simulink model "VCUSTM32"  (R2024b)
settings: Solver=FixedStepDiscrete  StartTime=0.0  StopTime=1  FixedStep=0.001  RelTol=1e-3  EnableMultiTasking=on
libraries: stm32blockslib x16, simulink x4, canmsglib x3, stm32f4xxblockslib x2, stm32h7xxblockslib x1
settings Model: STM32="{\"DigitalPortRead\":[{\"ID\":\"CANTestingSTM32:620\"},{\"ID\":\"VCUSTM32:620\"}],\"SPIControllerTransfer\":[{\"ID\":\"CANTestingSTM32:616\"},{\"ID\":\"CANTestingSTM32:631\"},{\"ID\":\"CANTestingSTM32:632\"},{\"ID\":\"CANTestingSTM32:633\"},{\"ID\":\"CANTestingSTM32:634\"},{\"ID\":\"CANTestingSTM32:635\"},{\"ID\":\"CANTestingSTM32:636\"},{\"ID\":\"CANTestingSTM32:637\"},{\"ID\":\"CANTestingSTM32:638\"},{\"ID\":\"CANTestingSTM32:653\"},{\"ID\":\"CANTestingSTM32:709\"},{\"ID\":\"CANTestingSTM32:716\"},{\"ID\":\"CANTestingSTM32:722\"},{\"ID\":\"CANTestingSTM32:728\"},{\"ID\":\"CANTestingSTM32:786\"},{\"ID\":\"CANTestingSTM32:787\"}],\"AnalogInputForH7\":[{\"ID\":\"CANTestingSTM32:731\"},{\"ID\":\"VCUSTM32:731\"}],\"DigitalPortWrite\":[{\"ID\":\"CANTestingSTM32:747\"},{\"ID\":\"VCUSTM32:747\"}]}"  Creator=will  LastModifiedBy=William
settings SolverCC: AlgebraicLoopSolver=TrustRegion
settings DataIOCC: ReturnWorkspaceOutputs=off
settings OptimizationCC: DefaultParameterBehavior=Inlined  EnhancedBackFolding=on  PassReuseOutputArgsAs=Individual arguments  ZeroExternalMemoryAtStartup=off  ZeroInternalMemoryAtStartup=off  MaxStackSize=512  OptimizeBlockOrder=speed  DifferentSizesBufferReuse=on  OptimizationCustomize=off  EfficientTunableParamExpr=on
settings DebuggingCC: ParameterTunabilityLossMsg=error  UnconnectedInputMsg=warning  UnconnectedOutputMsg=warning  UnconnectedLineMsg=warning  ArithmeticOperatorsInVariantConditions=warning
settings HardwareCC: ProdBitPerPointer=32  ProdBitPerSizeT=32  ProdBitPerPtrDiffT=32  ProdLargestAtomicInteger=Long  ProdLargestAtomicFloat=Double  ProdWordSize=32  ProdLongLongMode=on  ProdHWDeviceType=ARM Compatible->ARM Cortex-M
settings ModelReferenceCC: EnableRefExpFcnMdlSchedulingChecks=on
settings SFSimCC: MATLABDynamicMemAlloc=off  CustomCodeUndefinedFunction=UseInterfaceOnly
settings RTWCC: Description=Embedded Coder  SystemTargetFile=ert.tlc  HardwareBoard=STM32H7xx Based (Single-core)  TemplateMakefile=ert_default_tmf  CustomHeaderCode="#include \"stm32h7xx_ll_tim.h\""  CustomInitializer=LL_TIM_EnableCounter(TIM2);  Toolchain=GNU Tools for ARM Embedded Processors  GPUComputeCapability=3.5
settings CodeAppCC: ForceParamTrailComments=on  IgnoreCustomStorageClasses=off  OperatorAnnotations=on  SimulinkDataObjDesc=on  SFDataObjDesc=on  InsertBlockDesc=on
settings ERTTargetCC: TargetLangStandard=C99 (ISO)  CodeReplacementLibrary=ARM Cortex-M  ExtModeTransport=3  ExtModeStaticAlloc=on  ExtModeStaticAllocSize=2048  ExtModeMexFile=ext_xcp  ExtModeIntrfLevel=Level2 - Open

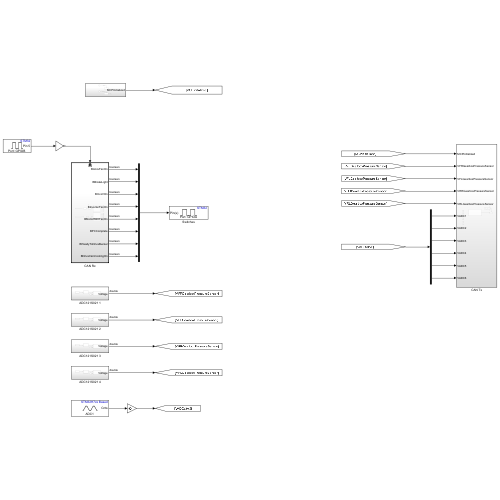
[thumbnail: Simulink's stored preview of the top-level diagram]
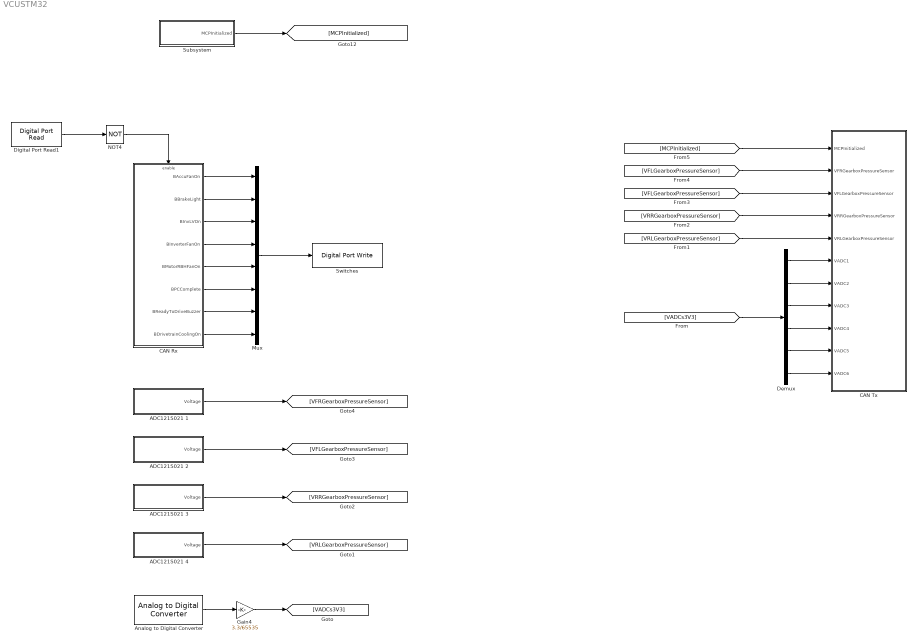
== system VCUSTM32 ==
  ADC121S021 1 : Subsystem
  ADC121S021 2 : Subsystem
  ADC121S021 3 : Subsystem
  ADC121S021 4 : Subsystem
  Analog to Digital Converter : stm32h7xxblockslib/Analog to Digital Converter  ADCModule=ADC1  ConversionGroup=Regular  TriggerMode=Trigger and read  NumberOfConversions=6  EnableBufferConv=off  BufferLength=1  OutputStatus=off  SampleTime=-1  EnableSimPort=off  hoistedMaskSrc=ECSoC/ECSimCodegen/Analog to Digital Converter
  CAN Rx : Subsystem  TreatAsAtomicUnit=on
  CAN Tx : Subsystem
  Demux : Demux  Outputs=6
  Digital Port Read1 : stm32f4xxblockslib/Digital Port Read  PortName=GPIOB  PinNumber=5  ReadOperation=on  IOAsArray=off  SampleTime=-1  EnableSimPort=off  hoistedMaskSrc=ECSoC/ECSimCodegen/Digital Port Read
      settings: LibrarySourceBlock=stm32f2xxblockslib/Digital Port Read
  Gain4 : Gain  Gain=3.3/65535  OutDataTypeStr=single
  Mux : Mux  Inputs=8
  NOT4 : Logic  Operator=NOT  IconShape=distinctive  AllPortsSameDT=off  OutDataTypeStr=boolean
  Subsystem : Subsystem
  Switches : stm32f4xxblockslib/Digital Port Write  PortName=GPIOA  PinNumber=[0, 1, 2, 3, 4]  ReadOperation=off  IOAsArray=on  EnableSimPort=off  hoistedMaskSrc=ECSoC/ECSimCodegen/Digital Port Write
      settings: LibrarySourceBlock=stm32h7xxblockslib/Digital Port Write
  wires:
  Subsystem/1(MCPInitialized) -> [MCPInitialized]
  NOT4/1 -> CAN Rx/Enable
  Digital Port Read1/1 -> NOT4/1
  Analog to Digital Converter/1 -> Gain4/1
  CAN Rx/6(BPCComplete) -> Mux/6
  CAN Rx/5(BMotorRBHFanOn) -> Mux/5
  CAN Rx/4(BInverterFanOn) -> Mux/4
  CAN Rx/3(BInvLVOn) -> Mux/3
  CAN Rx/2(BBrakeLight) -> Mux/2
  CAN Rx/1(BAccuFanOn) -> Mux/1
  CAN Rx/7(BReadyToDriveBuzzer) -> Mux/7
  CAN Rx/8(BDrivetrainCoolingOn) -> Mux/8
  Mux/1 -> Switches/1
  Gain4/1 -> [VADCs3V3]
  Demux/6 -> CAN Tx/11(VADC6)
  Demux/5 -> CAN Tx/10(VADC5)
  Demux/4 -> CAN Tx/9(VADC4)
  Demux/3 -> CAN Tx/8(VADC3)
  Demux/2 -> CAN Tx/7(VADC2)
  Demux/1 -> CAN Tx/6(VADC1)
  [VADCs3V3] -> Demux/1
  ADC121S021 1/1(Voltage) -> [VFRGearboxPressureSensor]
  ADC121S021 2/1(Voltage) -> [VFLGearboxPressureSensor]
  ADC121S021 3/1(Voltage) -> [VRRGearboxPressureSensor]
  ADC121S021 4/1(Voltage) -> [VRLGearboxPressureSensor]
  [VFLGearboxPressureSensor] -> CAN Tx/2(VFRGearboxPressureSensor)
  [VFLGearboxPressureSensor] -> CAN Tx/3(VFLGearboxPressureSensor)
  [VRRGearboxPressureSensor] -> CAN Tx/4(VRRGearboxPressureSensor)
  [VRLGearboxPressureSensor] -> CAN Tx/5(VRLGearboxPressureSensor)
  [MCPInitialized] -> CAN Tx/1(MCPInitialized)

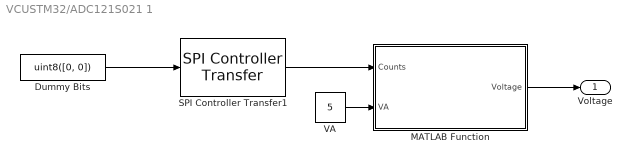
== system VCUSTM32/ADC121S021 1 ==
  Dummy Bits : Constant  Value=uint8([0, 0])
  MATLAB Function : MATLAB Function  TreatAsAtomicUnit=on
  SPI Controller Transfer1 : stm32blockslib/SPI Controller Transfer  Priority=2  SPIModuleSelect=SPI1  ClockPolarity=Low  ClockPhase=1 Edge  SPIModule=uint32(0)  Mode=Master  BusSpeed=uint32(1000000)  FirstBitToTransfer=Most significant bit (MSB)  ClockMode=0  BlockFunction=Transfer  EnableRegisterAddress=off  RegisterAddress=0  OutputDataType=uint8  OutputDataLength=1  OutputStatus=off  BlockingMode=on  Timeout=0.01  DataBits=8  UseCustomSSPin=Explicit GPIO calls  ActiveLowSSPin=Active low  Port_Select=GPIOA  Pin=4
      settings: LibrarySourceBlock=stm32h7xxblockslib/SPI Controller Transfer
  VA : Constant  Value=5
  Voltage : Outport  OutDataTypeStr=double
  wires:
  Dummy Bits/1 -> SPI Controller Transfer1/1
  SPI Controller Transfer1/1 -> MATLAB Function/1(Counts)
  VA/1 -> MATLAB Function/2(VA)
  MATLAB Function/1(Voltage) -> Voltage/1

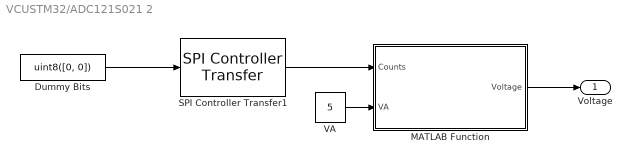
== system VCUSTM32/ADC121S021 2 ==
  Dummy Bits : Constant  Value=uint8([0, 0])
  MATLAB Function : MATLAB Function  TreatAsAtomicUnit=on
  SPI Controller Transfer1 : stm32blockslib/SPI Controller Transfer  Priority=2  SPIModuleSelect=SPI1  ClockPolarity=Low  ClockPhase=1 Edge  SPIModule=uint32(0)  Mode=Master  BusSpeed=uint32(1000000)  FirstBitToTransfer=Most significant bit (MSB)  ClockMode=0  BlockFunction=Transfer  EnableRegisterAddress=off  RegisterAddress=0  OutputDataType=uint8  OutputDataLength=1  OutputStatus=off  BlockingMode=on  Timeout=0.01  DataBits=8  UseCustomSSPin=Explicit GPIO calls  ActiveLowSSPin=Active low  Port_Select=GPIOA  Pin=4
      settings: LibrarySourceBlock=stm32h7xxblockslib/SPI Controller Transfer
  VA : Constant  Value=5
  Voltage : Outport  OutDataTypeStr=double
  wires:
  Dummy Bits/1 -> SPI Controller Transfer1/1
  SPI Controller Transfer1/1 -> MATLAB Function/1(Counts)
  VA/1 -> MATLAB Function/2(VA)
  MATLAB Function/1(Voltage) -> Voltage/1

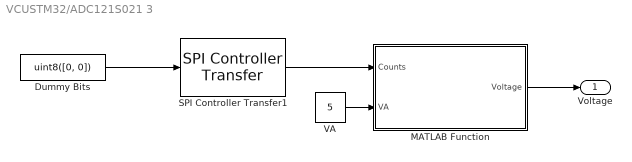
== system VCUSTM32/ADC121S021 3 ==
  Dummy Bits : Constant  Value=uint8([0, 0])
  MATLAB Function : MATLAB Function  TreatAsAtomicUnit=on
  SPI Controller Transfer1 : stm32blockslib/SPI Controller Transfer  Priority=2  SPIModuleSelect=SPI1  ClockPolarity=Low  ClockPhase=1 Edge  SPIModule=uint32(0)  Mode=Master  BusSpeed=uint32(1000000)  FirstBitToTransfer=Most significant bit (MSB)  ClockMode=0  BlockFunction=Transfer  EnableRegisterAddress=off  RegisterAddress=0  OutputDataType=uint8  OutputDataLength=1  OutputStatus=off  BlockingMode=on  Timeout=0.01  DataBits=8  UseCustomSSPin=Explicit GPIO calls  ActiveLowSSPin=Active low  Port_Select=GPIOA  Pin=4
      settings: LibrarySourceBlock=stm32h7xxblockslib/SPI Controller Transfer
  VA : Constant  Value=5
  Voltage : Outport  OutDataTypeStr=double
  wires:
  Dummy Bits/1 -> SPI Controller Transfer1/1
  SPI Controller Transfer1/1 -> MATLAB Function/1(Counts)
  VA/1 -> MATLAB Function/2(VA)
  MATLAB Function/1(Voltage) -> Voltage/1

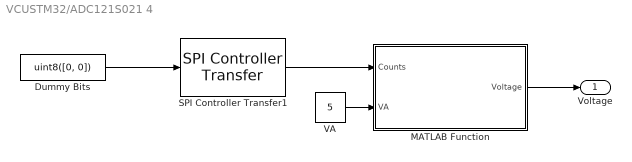
== system VCUSTM32/ADC121S021 4 ==
  Dummy Bits : Constant  Value=uint8([0, 0])
  MATLAB Function : MATLAB Function  TreatAsAtomicUnit=on
  SPI Controller Transfer1 : stm32blockslib/SPI Controller Transfer  Priority=2  SPIModuleSelect=SPI1  ClockPolarity=Low  ClockPhase=1 Edge  SPIModule=uint32(0)  Mode=Master  BusSpeed=uint32(1000000)  FirstBitToTransfer=Most significant bit (MSB)  ClockMode=0  BlockFunction=Transfer  EnableRegisterAddress=off  RegisterAddress=0  OutputDataType=uint8  OutputDataLength=1  OutputStatus=off  BlockingMode=on  Timeout=0.01  DataBits=8  UseCustomSSPin=Explicit GPIO calls  ActiveLowSSPin=Active low  Port_Select=GPIOA  Pin=4
      settings: LibrarySourceBlock=stm32h7xxblockslib/SPI Controller Transfer
  VA : Constant  Value=5
  Voltage : Outport  OutDataTypeStr=double
  wires:
  Dummy Bits/1 -> SPI Controller Transfer1/1
  SPI Controller Transfer1/1 -> MATLAB Function/1(Counts)
  VA/1 -> MATLAB Function/2(VA)
  MATLAB Function/1(Voltage) -> Voltage/1

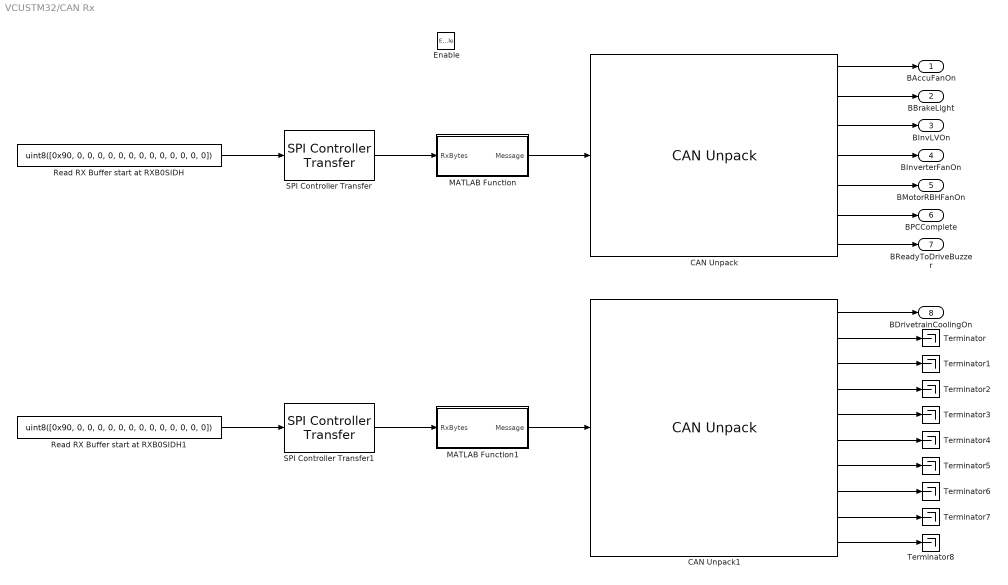
== system VCUSTM32/CAN Rx ==
  Enable : EnablePort
  CAN Unpack : canmsglib/CAN Unpack  CANdbFile=C:\Users\will\Desktop\STM32Projects\PDUSTM32\CAN3_26.05.26.dbc  MsgList=ETAS_0x603  MsgName=ETAS_0x603  MsgIDType=Standard (11-bit identifier)  MsgIdentifier=1539  MsgLength=8  SignalInfo={'BAccuFanOn','24','8','LE','unsigned','Standard','0','1','0','0','255';'BBrakeLight','0','8','LE','unsigned','Standard','0','1','0','0','255';'BInvLVOn','32','8','LE','unsigned','Standard','0','1','0','0','255';'BInverterFanOn','8','8','LE','unsigned','Standard','0','1','0','0','255';'BMotorRBHFanOn','16','8','LE','unsigned','Standard','0','1','0','0','255';'BPCComplete','40','8','LE','unsigned','Standard','0','1','0','0','255';'BReadyToDriveBuzzer','48','8','LE','unsigned','Standard','0','1','0','0','255'}  IDPort=off  TimestampPort=off  ErrorPort=off  RemotePort=off  LengthPort=off  StatusPort=off  ApplyMinMax=off
      settings: LibrarySourceBlock=stmutilitieslib/CAN Unpack  DataFormat=CANdb specified signals
  CAN Unpack1 : canmsglib/CAN Unpack  CANdbFile=C:\Users\will\Desktop\STM32Projects\PDUSTM32\CAN3_26.05.26.dbc  MsgList=ETAS_0x519  MsgName=ETAS_0x519  MsgIDType=Standard (11-bit identifier)  MsgIdentifier=1305  MsgLength=8  SignalInfo={'BDrivetrainCoolingOn','52','1','LE','unsigned','Standard','0','1','0','0','1';'BTCOn','51','1','LE','unsigned','Standard','0','1','0','0','1';'BTVOn','50','1','LE','unsigned','Standard','0','1','0','0','1';'NABSDTermFL','10','5','LE','unsigned','Standard','0','0.1','-3.1','-3.1','0';'NABSDTermFR','15','5','LE','unsigned','Standard','0','0.1','-3.1','-3.1','0';'NABSPTermRL','0','5','LE','unsigned','Standard','0','0.1','-3.1','-3.1','0';'NABSPTermRR','5','5','LE','unsigned','Standard','0','0.1','-3.1','-3.1','0';'PHighCellTempDischargeDerate','40','10','LE','unsigned','Standard','0','0.1','0','0','102.3';'PHighCellTempRegenDerate','30','10','LE','unsigned','Standard','0','0.1','-100','-100','0';'PRegenDerate','20','10','LE','unsigned','Standard','0','0.1','0','0','102.3'}  IDPort=off  TimestampPort=off  ErrorPort=off  RemotePort=off  LengthPort=off  StatusPort=off  ApplyMinMax=off
      settings: LibrarySourceBlock=stmutilitieslib/CAN Unpack  DataFormat=CANdb specified signals
  MATLAB Function : MATLAB Function  TreatAsAtomicUnit=on
  MATLAB Function1 : MATLAB Function  TreatAsAtomicUnit=on
  Read RX Buffer start at RXB0SIDH : Constant  Value=uint8([0x90, 0, 0, 0, 0, 0, 0, 0, 0, 0, 0, 0, 0, 0])
  Read RX Buffer start at RXB0SIDH1 : Constant  Value=uint8([0x90, 0, 0, 0, 0, 0, 0, 0, 0, 0, 0, 0, 0, 0])
  SPI Controller Transfer : stm32blockslib/SPI Controller Transfer  Priority=1  SPIModuleSelect=SPI1  ClockPolarity=Low  ClockPhase=1 Edge  SPIModule=uint32(0)  Mode=Master  BusSpeed=uint32(1000000)  FirstBitToTransfer=Most significant bit (MSB)  ClockMode=0  BlockFunction=Transfer  EnableRegisterAddress=off  RegisterAddress=0  OutputDataType=uint8  OutputDataLength=1  OutputStatus=off  BlockingMode=on  Timeout=0.01  DataBits=8  UseCustomSSPin=Explicit GPIO calls  ActiveLowSSPin=Active low  Port_Select=GPIOA  Pin=4
      settings: LibrarySourceBlock=stm32h7xxblockslib/SPI Controller Transfer
  SPI Controller Transfer1 : stm32blockslib/SPI Controller Transfer  Priority=2  SPIModuleSelect=SPI1  ClockPolarity=Low  ClockPhase=1 Edge  SPIModule=uint32(0)  Mode=Master  BusSpeed=uint32(1000000)  FirstBitToTransfer=Most significant bit (MSB)  ClockMode=0  BlockFunction=Transfer  EnableRegisterAddress=off  RegisterAddress=0  OutputDataType=uint8  OutputDataLength=1  OutputStatus=off  BlockingMode=on  Timeout=0.01  DataBits=8  UseCustomSSPin=Explicit GPIO calls  ActiveLowSSPin=Active low  Port_Select=GPIOA  Pin=4
      settings: LibrarySourceBlock=stm32h7xxblockslib/SPI Controller Transfer
  Terminator{,1..8} (9 alike) : Terminator
  BAccuFanOn : Outport  OutDataTypeStr=boolean
  BBrakeLight : Outport  Port=2  OutDataTypeStr=boolean
  BInvLVOn : Outport  Port=3  OutDataTypeStr=boolean
  BInverterFanOn : Outport  Port=4  OutDataTypeStr=boolean
  BMotorRBHFanOn : Outport  Port=5  OutDataTypeStr=boolean
  BPCComplete : Outport  Port=6  OutDataTypeStr=boolean
  BReadyToDriveBuzzer : Outport  Port=7  OutDataTypeStr=boolean
  BDrivetrainCoolingOn : Outport  Port=8  OutDataTypeStr=boolean
  wires:
  Read RX Buffer start at RXB0SIDH/1 -> SPI Controller Transfer/1
  SPI Controller Transfer/1 -> MATLAB Function/1(RxBytes)
  MATLAB Function/1(Message) -> CAN Unpack/1
  SPI Controller Transfer1/1 -> MATLAB Function1/1(RxBytes)
  MATLAB Function1/1(Message) -> CAN Unpack1/1
  Read RX Buffer start at RXB0SIDH1/1 -> SPI Controller Transfer1/1
  CAN Unpack/1 -> BAccuFanOn/1
  CAN Unpack/2 -> BBrakeLight/1
  CAN Unpack/3 -> BInvLVOn/1
  CAN Unpack1/1 -> BDrivetrainCoolingOn/1
  CAN Unpack/4 -> BInverterFanOn/1
  CAN Unpack/5 -> BMotorRBHFanOn/1
  CAN Unpack/6 -> BPCComplete/1
  CAN Unpack/7 -> BReadyToDriveBuzzer/1
  CAN Unpack1/2 -> Terminator/1
  CAN Unpack1/3 -> Terminator1/1
  CAN Unpack1/4 -> Terminator2/1
  CAN Unpack1/5 -> Terminator3/1
  CAN Unpack1/6 -> Terminator4/1
  CAN Unpack1/7 -> Terminator5/1
  CAN Unpack1/8 -> Terminator6/1
  CAN Unpack1/9 -> Terminator7/1
  CAN Unpack1/10 -> Terminator8/1

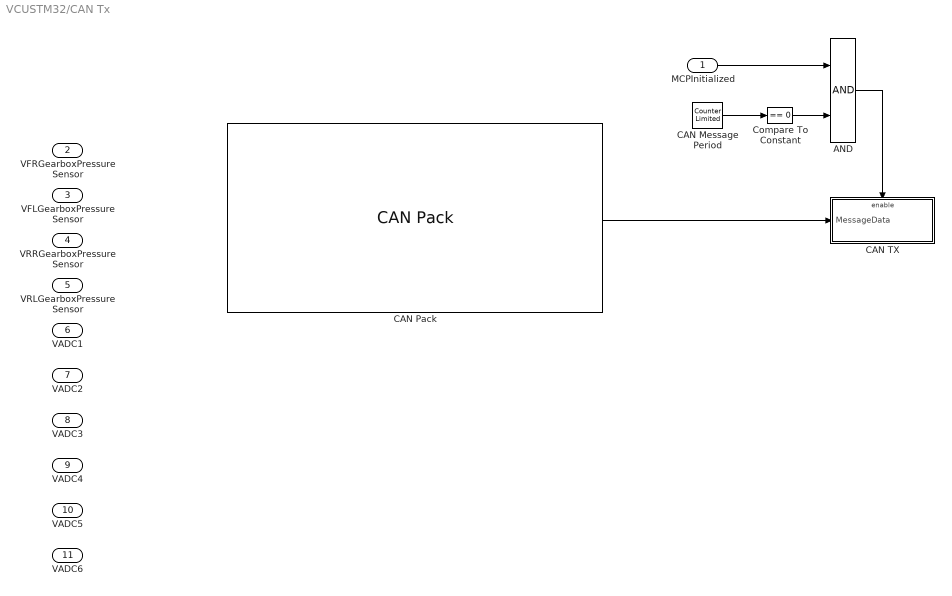
== system VCUSTM32/CAN Tx ==
  MCPInitialized : Inport
  VFRGearboxPressureSensor : Inport  Port=2
  VFLGearboxPressureSensor : Inport  Port=3
  VRRGearboxPressureSensor : Inport  Port=4
  VRLGearboxPressureSensor : Inport  Port=5
  VADC1 : Inport  Port=6
  VADC2 : Inport  Port=7
  VADC3 : Inport  Port=8
  VADC4 : Inport  Port=9
  VADC5 : Inport  Port=10
  VADC6 : Inport  Port=11
  AND : Logic  IconShape=distinctive  AllPortsSameDT=off  OutDataTypeStr=boolean
  CAN Message Period : simulink/Sources/Counter Limited  uplimit=10  tsamp=-1
  CAN Pack : canmsglib/CAN Pack  CANdbFile=C:\Users\will\Desktop\STM32Projects\PDUSTM32\CAN3_26.05.26.dbc  MsgList=PDM_0x500  MsgName=PDM_0x500  MsgIDType=Standard (11-bit identifier)  MsgIdentifier=1280  CANIDInput=off  MsgLength=8  Remote=off  ApplyMinMax=off  BusOutput=on  SignalInfo={'IPDM','16','8','LE','unsigned','Standard','0','1','0','0','255';'NDeviceError','24','8','LE','unsigned','Standard','0','1','0','0','255';'TPDM','8','8','LE','unsigned','Standard','0','1','0','0','255';'VPDM','0','8','LE','unsigned','Standard','0','1','0','0','255'}
      settings: LibrarySourceBlock=stmutilitieslib/CAN Pack  DataFormat=CANdb specified signals
  CAN TX : Subsystem  TreatAsAtomicUnit=on
  Compare To Constant : simulink/Logic and Bit Operations/Compare To Constant  relop===  const=0  OutDataTypeStr=boolean
  wires:
  AND/1 -> CAN TX/Enable
  CAN Pack/1 -> CAN TX/1(MessageData)
  CAN Message Period/1 -> Compare To Constant/1
  MCPInitialized/1 -> AND/1
  Compare To Constant/1 -> AND/2

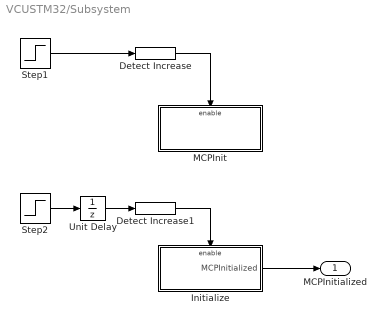
== system VCUSTM32/Subsystem ==
  Detect Increase : simulink/Logic and Bit Operations/Detect Increase  vinit=0.0  OutDataTypeStr=boolean
  Detect Increase1 : simulink/Logic and Bit Operations/Detect Increase  vinit=0.0  OutDataTypeStr=boolean
  Initialize : Subsystem  TreatAsAtomicUnit=on
  MCPInit : Subsystem  TreatAsAtomicUnit=on
  Step1 : Step
  Step2 : Step
  Unit Delay : UnitDelay  SampleTime=-1  HasFrameUpgradeWarning=on
  MCPInitialized : Outport
  wires:
  Step1/1 -> Detect Increase/1
  Unit Delay/1 -> Detect Increase1/1
  Detect Increase1/1 -> Initialize/Enable
  Detect Increase/1 -> MCPInit/Enable
  Step2/1 -> Unit Delay/1
  Initialize/1(MCPInitialized) -> MCPInitialized/1

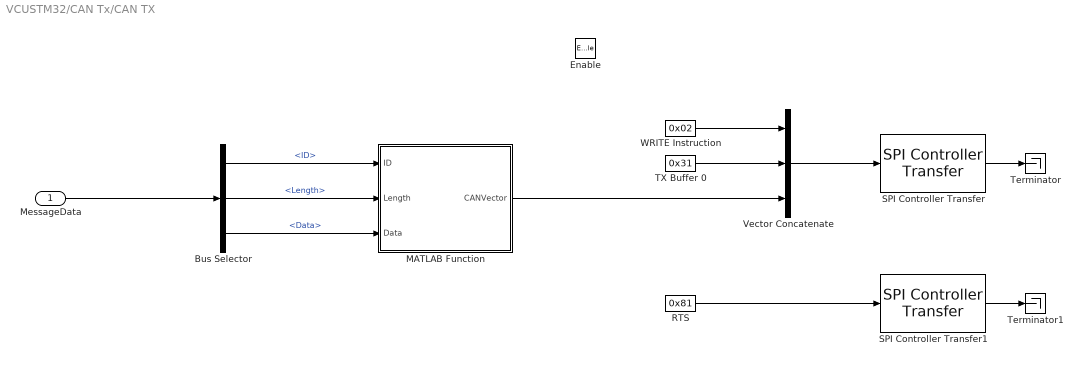
== system VCUSTM32/CAN Tx/CAN TX ==
  MessageData : Inport
  Enable : EnablePort
  Bus Selector : BusSelector  OutputSignals=ID,Length,Data
  MATLAB Function : MATLAB Function  TreatAsAtomicUnit=on
  RTS : Constant  Value=0x81  OutDataTypeStr=uint8  SampleTime=-1
  SPI Controller Transfer : stm32blockslib/SPI Controller Transfer  Priority=1  SPIModuleSelect=SPI1  ClockPolarity=Low  ClockPhase=1 Edge  SPIModule=uint32(0)  Mode=Master  BusSpeed=uint32(1000000)  FirstBitToTransfer=Most significant bit (MSB)  ClockMode=0  BlockFunction=Transfer  EnableRegisterAddress=off  RegisterAddress=0  OutputDataType=uint8  OutputDataLength=1  OutputStatus=off  BlockingMode=on  Timeout=0.01  DataBits=8  UseCustomSSPin=Explicit GPIO calls  ActiveLowSSPin=Active low  Port_Select=GPIOA  Pin=4
      settings: LibrarySourceBlock=stm32h7xxblockslib/SPI Controller Transfer
  SPI Controller Transfer1 : stm32blockslib/SPI Controller Transfer  Priority=5  SPIModuleSelect=SPI1  ClockPolarity=Low  ClockPhase=1 Edge  SPIModule=uint32(0)  Mode=Master  BusSpeed=uint32(1000000)  FirstBitToTransfer=Most significant bit (MSB)  ClockMode=0  BlockFunction=Transfer  EnableRegisterAddress=off  RegisterAddress=0  OutputDataType=uint8  OutputDataLength=1  OutputStatus=off  BlockingMode=on  Timeout=0.01  DataBits=8  UseCustomSSPin=Explicit GPIO calls  ActiveLowSSPin=Active low  Port_Select=GPIOA  Pin=4
      settings: LibrarySourceBlock=stm32h7xxblockslib/SPI Controller Transfer
  TX Buffer 0 : Constant  Value=0x31  OutDataTypeStr=uint8  SampleTime=-1
  Terminator : Terminator
  Terminator1 : Terminator
  Vector Concatenate : Concatenate  NumInputs=3
  WRITE Instruction : Constant  Value=0x02  OutDataTypeStr=uint8  SampleTime=-1
  wires:
  SPI Controller Transfer1/1 -> Terminator1/1
  Bus Selector/2 -> MATLAB Function/2(Length)  "<Length>"
  Bus Selector/1 -> MATLAB Function/1(ID)  "<ID>"
  MATLAB Function/1(CANVector) -> Vector Concatenate/3
  TX Buffer 0/1 -> Vector Concatenate/2
  Bus Selector/3 -> MATLAB Function/3(Data)  "<Data>"
  MessageData/1 -> Bus Selector/1
  WRITE Instruction/1 -> Vector Concatenate/1
  SPI Controller Transfer/1 -> Terminator/1
  Vector Concatenate/1 -> SPI Controller Transfer/1
  RTS/1 -> SPI Controller Transfer1/1

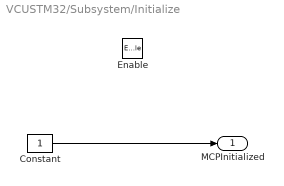
== system VCUSTM32/Subsystem/Initialize ==
  Enable : EnablePort
  Constant : Constant  OutDataTypeStr=boolean
  MCPInitialized : Outport
  wires:
  Constant/1 -> MCPInitialized/1

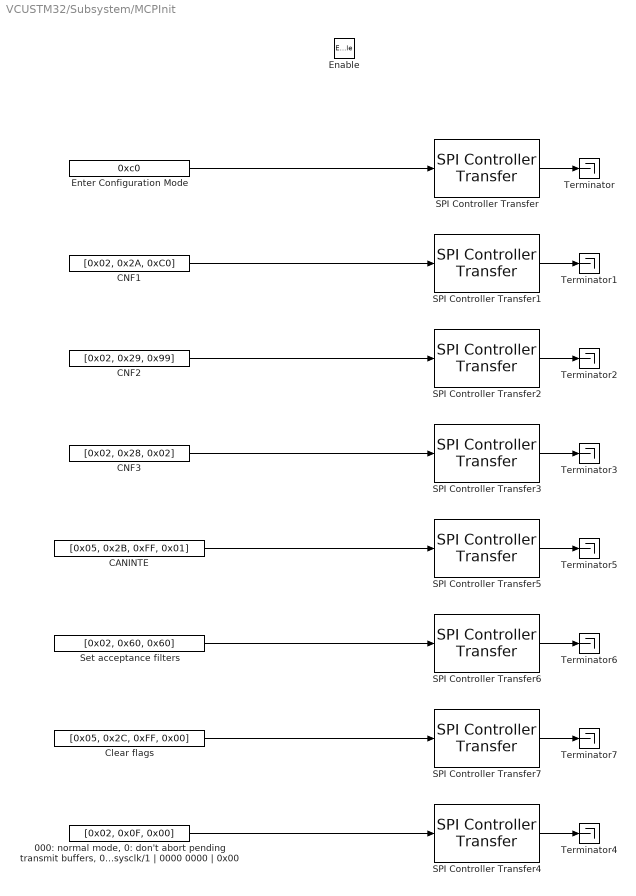
== system VCUSTM32/Subsystem/MCPInit ==
  Enable : EnablePort
  " 000: normal mode, 0: don't abort pending transmit buffers, 0: one-shot disabled, 0: CLKOUT disabled, 00: sysclk/1 | 0000 0000 | 0x00" : Constant  Value=[0x02, 0x0F, 0x00]  OutDataTypeStr=uint8
  CANINTE : Constant  Value=[0x05, 0x2B, 0xFF, 0x01]  OutDataTypeStr=uint8
  CNF1 : Constant  Value=[0x02, 0x2A, 0xC0]  OutDataTypeStr=uint8
  CNF2 : Constant  Value=[0x02, 0x29, 0x99]  OutDataTypeStr=uint8
  CNF3 : Constant  Value=[0x02, 0x28, 0x02]  OutDataTypeStr=uint8
  Clear flags : Constant  Value=[0x05, 0x2C, 0xFF, 0x00]  OutDataTypeStr=uint8
  Enter Configuration Mode : Constant  Value=0xc0  OutDataTypeStr=uint8
  SPI Controller Transfer : stm32blockslib/SPI Controller Transfer  Priority=3  SPIModuleSelect=SPI1  ClockPolarity=Low  ClockPhase=1 Edge  SPIModule=uint32(0)  Mode=Master  BusSpeed=uint32(1000000)  FirstBitToTransfer=Most significant bit (MSB)  ClockMode=0  BlockFunction=Transfer  EnableRegisterAddress=off  RegisterAddress=0  OutputDataType=uint8  OutputDataLength=1  OutputStatus=off  BlockingMode=on  Timeout=0.01  DataBits=8  UseCustomSSPin=Explicit GPIO calls  ActiveLowSSPin=Active low  Port_Select=GPIOA  Pin=4
      settings: LibrarySourceBlock=stm32h7xxblockslib/SPI Controller Transfer
  SPI Controller Transfer1 : stm32blockslib/SPI Controller Transfer  Priority=4  SPIModuleSelect=SPI1  ClockPolarity=Low  ClockPhase=1 Edge  SPIModule=uint32(0)  Mode=Master  BusSpeed=uint32(1000000)  FirstBitToTransfer=Most significant bit (MSB)  ClockMode=0  BlockFunction=Transfer  EnableRegisterAddress=off  RegisterAddress=0  OutputDataType=uint8  OutputDataLength=1  OutputStatus=off  BlockingMode=on  Timeout=0.01  DataBits=8  UseCustomSSPin=Explicit GPIO calls  ActiveLowSSPin=Active low  Port_Select=GPIOA  Pin=4
      settings: LibrarySourceBlock=stm32h7xxblockslib/SPI Controller Transfer
  SPI Controller Transfer2 : stm32blockslib/SPI Controller Transfer  Priority=5  SPIModuleSelect=SPI1  ClockPolarity=Low  ClockPhase=1 Edge  SPIModule=uint32(0)  Mode=Master  BusSpeed=uint32(1000000)  FirstBitToTransfer=Most significant bit (MSB)  ClockMode=0  BlockFunction=Transfer  EnableRegisterAddress=off  RegisterAddress=0  OutputDataType=uint8  OutputDataLength=1  OutputStatus=off  BlockingMode=on  Timeout=0.01  DataBits=8  UseCustomSSPin=Explicit GPIO calls  ActiveLowSSPin=Active low  Port_Select=GPIOA  Pin=4
      settings: LibrarySourceBlock=stm32h7xxblockslib/SPI Controller Transfer
  SPI Controller Transfer3 : stm32blockslib/SPI Controller Transfer  Priority=6  SPIModuleSelect=SPI1  ClockPolarity=Low  ClockPhase=1 Edge  SPIModule=uint32(0)  Mode=Master  BusSpeed=uint32(1000000)  FirstBitToTransfer=Most significant bit (MSB)  ClockMode=0  BlockFunction=Transfer  EnableRegisterAddress=off  RegisterAddress=0  OutputDataType=uint8  OutputDataLength=1  OutputStatus=off  BlockingMode=on  Timeout=0.01  DataBits=8  UseCustomSSPin=Explicit GPIO calls  ActiveLowSSPin=Active low  Port_Select=GPIOA  Pin=4
      settings: LibrarySourceBlock=stm32h7xxblockslib/SPI Controller Transfer
  SPI Controller Transfer4 : stm32blockslib/SPI Controller Transfer  Priority=10  SPIModuleSelect=SPI1  ClockPolarity=Low  ClockPhase=1 Edge  SPIModule=uint32(0)  Mode=Master  BusSpeed=uint32(1000000)  FirstBitToTransfer=Most significant bit (MSB)  ClockMode=0  BlockFunction=Transfer  EnableRegisterAddress=off  RegisterAddress=0  OutputDataType=uint8  OutputDataLength=1  OutputStatus=off  BlockingMode=on  Timeout=0.01  DataBits=8  UseCustomSSPin=Explicit GPIO calls  ActiveLowSSPin=Active low  Port_Select=GPIOA  Pin=4
      settings: LibrarySourceBlock=stm32h7xxblockslib/SPI Controller Transfer
  SPI Controller Transfer5 : stm32blockslib/SPI Controller Transfer  Priority=7  SPIModuleSelect=SPI1  ClockPolarity=Low  ClockPhase=1 Edge  SPIModule=uint32(0)  Mode=Master  BusSpeed=uint32(1000000)  FirstBitToTransfer=Most significant bit (MSB)  ClockMode=0  BlockFunction=Transfer  EnableRegisterAddress=off  RegisterAddress=0  OutputDataType=uint8  OutputDataLength=1  OutputStatus=off  BlockingMode=on  Timeout=0.01  DataBits=8  UseCustomSSPin=Explicit GPIO calls  ActiveLowSSPin=Active low  Port_Select=GPIOA  Pin=4
      settings: LibrarySourceBlock=stm32h7xxblockslib/SPI Controller Transfer
  SPI Controller Transfer6 : stm32blockslib/SPI Controller Transfer  Priority=8  SPIModuleSelect=SPI1  ClockPolarity=Low  ClockPhase=1 Edge  SPIModule=uint32(0)  Mode=Master  BusSpeed=uint32(1000000)  FirstBitToTransfer=Most significant bit (MSB)  ClockMode=0  BlockFunction=Transfer  EnableRegisterAddress=off  RegisterAddress=0  OutputDataType=uint8  OutputDataLength=1  OutputStatus=off  BlockingMode=on  Timeout=0.01  DataBits=8  UseCustomSSPin=Explicit GPIO calls  ActiveLowSSPin=Active low  Port_Select=GPIOA  Pin=4
      settings: LibrarySourceBlock=stm32h7xxblockslib/SPI Controller Transfer
  SPI Controller Transfer7 : stm32blockslib/SPI Controller Transfer  Priority=9  SPIModuleSelect=SPI1  ClockPolarity=Low  ClockPhase=1 Edge  SPIModule=uint32(0)  Mode=Master  BusSpeed=uint32(1000000)  FirstBitToTransfer=Most significant bit (MSB)  ClockMode=0  BlockFunction=Transfer  EnableRegisterAddress=off  RegisterAddress=0  OutputDataType=uint8  OutputDataLength=1  OutputStatus=off  BlockingMode=on  Timeout=0.01  DataBits=8  UseCustomSSPin=Explicit GPIO calls  ActiveLowSSPin=Active low  Port_Select=GPIOA  Pin=4
      settings: LibrarySourceBlock=stm32h7xxblockslib/SPI Controller Transfer
  Set acceptance filters : Constant  Value=[0x02, 0x60, 0x60]  OutDataTypeStr=uint8
  Terminator{,1..7} (8 alike) : Terminator
  wires:
  SPI Controller Transfer2/1 -> Terminator2/1
  Enter Configuration Mode/1 -> SPI Controller Transfer/1
  SPI Controller Transfer7/1 -> Terminator7/1
  Set acceptance filters/1 -> SPI Controller Transfer6/1
  SPI Controller Transfer3/1 -> Terminator3/1
  CANINTE/1 -> SPI Controller Transfer5/1
  CNF1/1 -> SPI Controller Transfer1/1
  SPI Controller Transfer6/1 -> Terminator6/1
  SPI Controller Transfer4/1 -> Terminator4/1
  CNF3/1 -> SPI Controller Transfer3/1
  SPI Controller Transfer/1 -> Terminator/1
  CNF2/1 -> SPI Controller Transfer2/1
  " 000: normal mode, 0: don't abort pending transmit buffers, 0: one-shot disabled, 0: CLKOUT disabled, 00: sysclk/1 | 0000 0000 | 0x00"/1 -> SPI Controller Transfer4/1
  SPI Controller Transfer5/1 -> Terminator5/1
  Clear flags/1 -> SPI Controller Transfer7/1
  SPI Controller Transfer1/1 -> Terminator1/1

== matlab function VCUSTM32/ADC121S021 1/MATLAB Function ==
  data: Counts input int8; Voltage output double; VA input double
function Voltage = ConvertToVoltage(Counts, VA)
    raw = uint16(Counts(1)) * 256 + uint16(Counts(2));
    counts = double(bitshift(raw, -1) & uint16(4095));
    Voltage = counts * (VA / 4095.0);
end

== matlab function VCUSTM32/CAN Rx/MATLAB Function ==
  data: RxBytes input uint8 size=14; Message output Bus: CAN_MESSAGE_def
function Message = DecodeCANMsg(RxBytes)
%#codegen

% rxBytes is uint8(1x14); byte 1 is the command echo (don't care)
SIDH = RxBytes(2);
SIDL = RxBytes(3);
EID8 = RxBytes(4);  %#ok — not used for standard frames
EID0 = RxBytes(5);  %#ok
DLC  = RxBytes(6);

% Assemble standard 11-bit ID
Message.ID       = uint32(bitor(uint32(bitshift(uint32(SIDH), 3)), ...
                            uint32(bitshift(uint32(SIDL), -5))));
Message.Extended = false;
Message.Remote   = false;
Message.Error    = false;
Message.Length   = double(bitand(DLC, uint8(15)));
Message.Data     = RxBytes(7:14);

== matlab function VCUSTM32/CAN Rx/MATLAB Function1 ==
  data: RxBytes input uint8 size=14; Message output Bus: CAN_MESSAGE_def
function Message = DecodeCANMsg(RxBytes)
%#codegen

% rxBytes is uint8(1x14); byte 1 is the command echo (don't care)
SIDH = RxBytes(2);
SIDL = RxBytes(3);
EID8 = RxBytes(4);  %#ok — not used for standard frames
EID0 = RxBytes(5);  %#ok
DLC  = RxBytes(6);

% Assemble standard 11-bit ID
Message.ID       = uint32(bitor(uint32(bitshift(uint32(SIDH), 3)), ...
                            uint32(bitshift(uint32(SIDL), -5))));
Message.Extended = false;
Message.Remote   = false;
Message.Error    = false;
Message.Length   = double(bitand(DLC, uint8(15)));
Message.Data     = RxBytes(7:14);

== matlab function VCUSTM32/ADC121S021 2/MATLAB Function ==
  data: Counts input int8; Voltage output double; VA input double
function Voltage = ConvertToVoltage(Counts, VA)
    raw = uint16(Counts(1)) * 256 + uint16(Counts(2));
    counts = double(bitshift(raw, -1) & uint16(4095));
    Voltage = counts * (VA / 4095.0);
end

== matlab function VCUSTM32/ADC121S021 3/MATLAB Function ==
  data: Counts input int8; Voltage output double; VA input double
function Voltage = ConvertToVoltage(Counts, VA)
    raw = uint16(Counts(1)) * 256 + uint16(Counts(2));
    counts = double(bitshift(raw, -1) & uint16(4095));
    Voltage = counts * (VA / 4095.0);
end

== matlab function VCUSTM32/ADC121S021 4/MATLAB Function ==
  data: Counts input int8; Voltage output double; VA input double
function Voltage = ConvertToVoltage(Counts, VA)
    raw = uint16(Counts(1)) * 256 + uint16(Counts(2));
    counts = double(bitshift(raw, -1) & uint16(4095));
    Voltage = counts * (VA / 4095.0);
end

== matlab function VCUSTM32/CAN Tx/CAN TX/MATLAB Function ==
  data: ID input uint32; CANVector output uint8; Length input uint8; Data input uint8
function CANVector = ConvertToVector(ID, Length, Data)
    %#codegen
    id_u16 = uint16(ID);
    len_u8 = uint8(Length);

    CANVector = zeros(1, 13, 'uint8');  % 13 bytes only — no instruction

    CANVector(1) = uint8(bitshift(id_u16, -3));              % SIDH: ID[10:3]
    CANVector(2) = uint8(bitshift(bitand(id_u16, uint16(7)), 5)); % SIDL: ID[2:0]<<5, EXIDE=0
    CANVector(3) = uint8(0);   % EID8 unused
    CANVector(4) = uint8(0);   % EID0 unused
    CANVector(5) = bitand(len_u8, uint8(15));  % DLC
    for i = 1:8
        CANVector(5+i) = uint8(Data(i));
    end
